simulink model "SIM_lqr_d"  (R2021b)
settings: Solver=VariableStepAuto  StartTime=0.0  StopTime=10.0  RelTol=1e-3
values from neighbouring files (symbols this model uses):
  a = sys_d.A    [LQR_controller.m]
  b = sys_d.B    [LQR_controller.m]
  c = sys_d.C    [LQR_controller.m]
  dd = sys_d.D    [LQR_controller.m]
  K = dlqr(a,b,Q,R)    [LQR_controller.m]
  x0 = [0,6]    [LQR_controller.m]
settings Model: Creator=kjnikhil  LastModifiedBy=kjnikhil

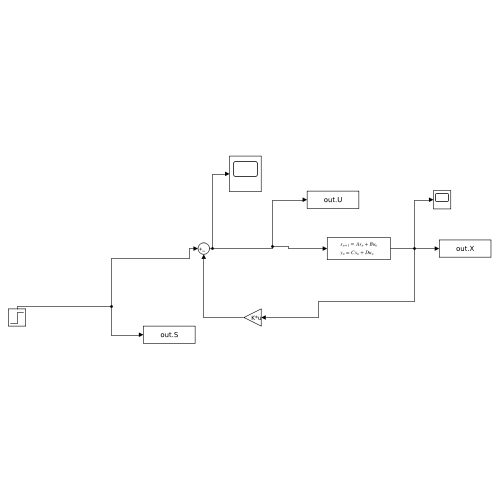
[thumbnail: Simulink's stored preview of the top-level diagram]
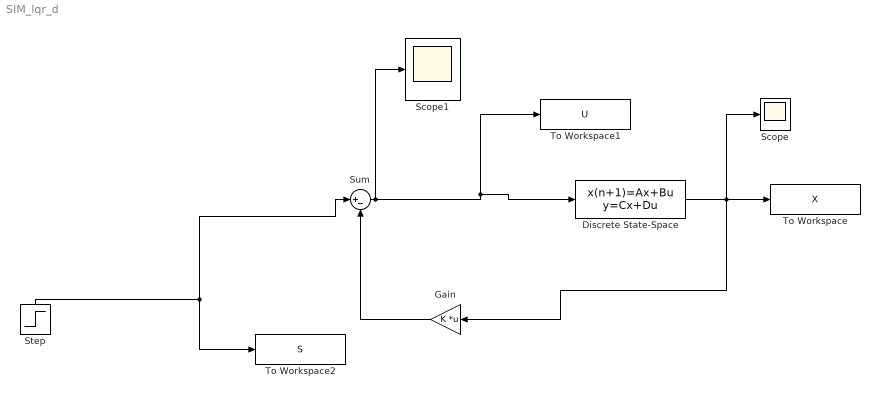
== system SIM_lqr_d ==
  Discrete State-Space : DiscreteStateSpace  A=a  B=b  C=c  D=dd  InitialCondition=x0  SampleTime=0.008
  Gain : Gain  Gain=K  Multiplication=Matrix(K*u)
  Scope : Scope
  Scope1 : Scope
  Step : Step  SampleTime=0
  Sum : Sum  Inputs=|+-
  To Workspace : ToWorkspace  VariableName=X  SaveFormat=Structure With Time  SampleTime=-1
  To Workspace1 : ToWorkspace  VariableName=U  SaveFormat=Structure With Time  SampleTime=-1
  To Workspace2 : ToWorkspace  VariableName=S  SaveFormat=Structure With Time  SampleTime=-1
  wires:
  Gain/1 -> Sum/2
  Step/1 -> To Workspace2/1, Sum/1
  Discrete State-Space/1 -> Gain/1, Scope/1, To Workspace/1
  Sum/1 -> Scope1/1, Discrete State-Space/1, To Workspace1/1
